simulink library "MAN_Library"  (R2023a)
settings: Solver=ode45  StartTime=0.0  StopTime=10.0  RelTol=1e-3  EnableMultiTasking=on
undefined symbols (not defined in the file): EventID
libraries: $bdroot x33, simulink_need_slupdate x1
(part 2 of 2)

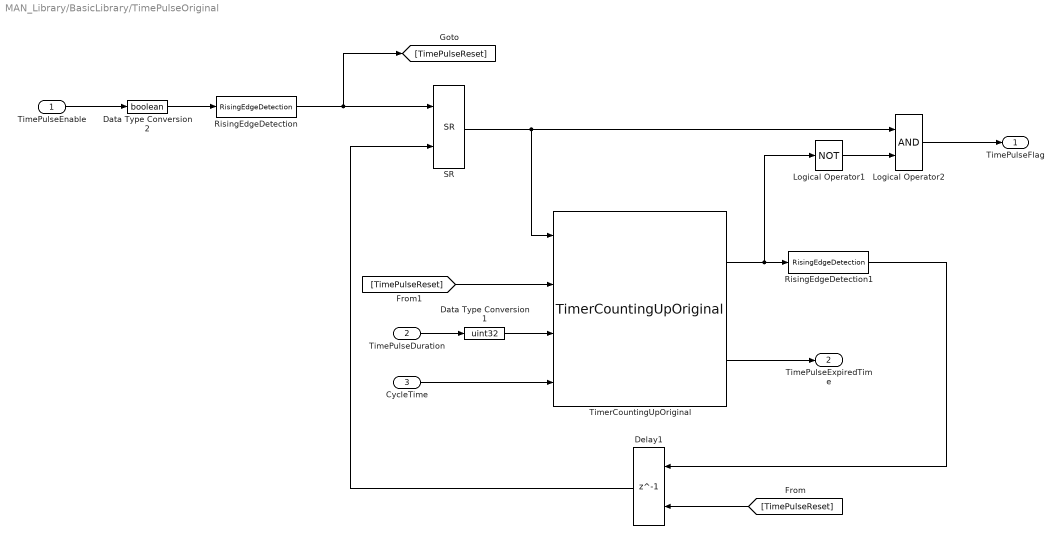
== system MAN_Library/BasicLibrary/TimePulseOriginal ==
  TimePulseEnable : Inport
  TimePulseDuration : Inport  Port=2
  CycleTime : Inport  Port=3
  Data Type Conversion1 : DataTypeConversion  OutDataTypeStr=uint32  SaturateOnIntegerOverflow=off  RndMeth=Floor
  Data Type Conversion2 : DataTypeConversion  OutDataTypeStr=boolean  SaturateOnIntegerOverflow=off  RndMeth=Floor
  Delay1 : Delay  DelayLength=1  InitialCondition=0  ExternalReset=Rising
      settings: InputPortMap=u0,r5
  Logical Operator1 : Logic  Operator=NOT  AllPortsSameDT=off  OutDataTypeStr=boolean
  Logical Operator2 : Logic  AllPortsSameDT=off  OutDataTypeStr=boolean
  RisingEdgeDetection : $bdroot/RisingEdgeDetection  SystemSampleTime=-1  VariantActivationTime=update diagram  Latency=0  AutoFrameSizeCalculation=off
  RisingEdgeDetection1 : $bdroot/RisingEdgeDetection  SystemSampleTime=-1  VariantActivationTime=update diagram  Latency=0  AutoFrameSizeCalculation=off
  SR : $bdroot/SR  SystemSampleTime=-1  VariantActivationTime=update diagram  Latency=0  AutoFrameSizeCalculation=off
  TimerCountingUpOriginal : $bdroot/BasicLibrary/TimerCountingUpOriginal  SystemSampleTime=-1  VariantActivationTime=update diagram  Latency=0  AutoFrameSizeCalculation=off
  TimePulseFlag : Outport
  TimePulseExpiredTime : Outport  Port=2
  wires:
  TimerCountingUpOriginal/2 -> TimePulseExpiredTime/1
  TimePulseDuration/1 -> Data Type Conversion1/1
  TimePulseEnable/1 -> Data Type Conversion2/1
  SR/1 -> TimerCountingUpOriginal/1, Logical Operator2/1
  TimerCountingUpOriginal/1 -> Logical Operator1/1, RisingEdgeDetection1/1
  RisingEdgeDetection1/1 -> Delay1/1
  Logical Operator2/1 -> TimePulseFlag/1
  Logical Operator1/1 -> Logical Operator2/2
  Data Type Conversion2/1 -> RisingEdgeDetection/1
  Data Type Conversion1/1 -> TimerCountingUpOriginal/3
  RisingEdgeDetection/1 -> [TimePulseReset], SR/1
  [TimePulseReset] -> Delay1/2
  [TimePulseReset] -> TimerCountingUpOriginal/2
  Delay1/1 -> SR/2
  CycleTime/1 -> TimerCountingUpOriginal/4

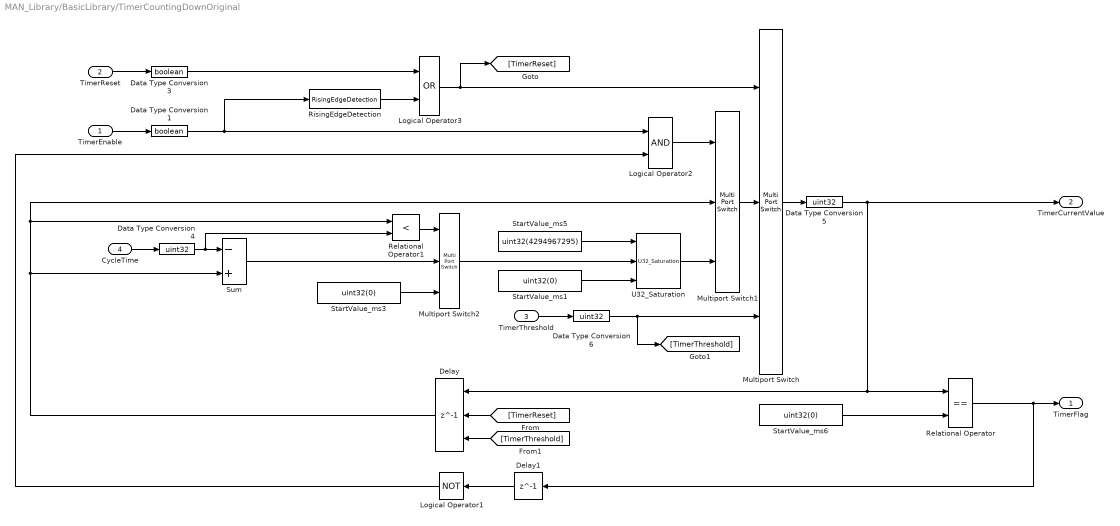
== system MAN_Library/BasicLibrary/TimerCountingDownOriginal ==
  TimerEnable : Inport
  TimerReset : Inport  Port=2
  TimerThreshold : Inport  Port=3
  CycleTime : Inport  Port=4
  Data Type Conversion1 : DataTypeConversion  OutDataTypeStr=boolean  SaturateOnIntegerOverflow=off  RndMeth=Floor
  Data Type Conversion3 : DataTypeConversion  OutDataTypeStr=boolean  SaturateOnIntegerOverflow=off  RndMeth=Floor
  Data Type Conversion4 : DataTypeConversion  OutDataTypeStr=uint32  SaturateOnIntegerOverflow=off  RndMeth=Floor
  Data Type Conversion5 : DataTypeConversion  OutDataTypeStr=uint32  SaturateOnIntegerOverflow=off  RndMeth=Floor
  Data Type Conversion6 : DataTypeConversion  OutDataTypeStr=uint32  SaturateOnIntegerOverflow=off  RndMeth=Floor
  Delay : Delay  DelayLength=1  InitialConditionSource=Input port  InitialCondition=0  ExternalReset=Rising
      settings: InputPortMap=u0,r5,p4
  Delay1 : Delay  DelayLength=1  InitialCondition=0
  Logical Operator1 : Logic  Operator=NOT  AllPortsSameDT=off  OutDataTypeStr=boolean
  Logical Operator2 : Logic  AllPortsSameDT=off  OutDataTypeStr=boolean
  Logical Operator3 : Logic  Operator=OR  AllPortsSameDT=off  OutDataTypeStr=boolean
  Multiport Switch : MultiPortSwitch  DataPortOrder=Zero-based contiguous  Inputs=2  zeroidx=on  SaturateOnIntegerOverflow=off  InputSameDT=off
  Multiport Switch1 : MultiPortSwitch  DataPortOrder=Zero-based contiguous  Inputs=2  zeroidx=on  SaturateOnIntegerOverflow=off  InputSameDT=off
  Multiport Switch2 : MultiPortSwitch  DataPortOrder=Zero-based contiguous  Inputs=2  zeroidx=on  SaturateOnIntegerOverflow=off  InputSameDT=off
  Relational Operator : RelationalOperator  Operator===  OutDataTypeStr=boolean  InputSameDT=off
  Relational Operator1 : RelationalOperator  Operator=<  OutDataTypeStr=boolean  InputSameDT=off
  RisingEdgeDetection : $bdroot/RisingEdgeDetection  SystemSampleTime=-1  VariantActivationTime=update diagram  Latency=0  AutoFrameSizeCalculation=off
  StartValue_ms1 : Constant  Value=uint32(0)  OutDataTypeStr=uint32
  StartValue_ms3 : Constant  Value=uint32(0)  OutDataTypeStr=uint32
  StartValue_ms5 : Constant  Value=uint32(4294967295)  OutDataTypeStr=uint32
  StartValue_ms6 : Constant  Value=uint32(0)  OutDataTypeStr=uint32
  Sum : Sum  Inputs=-+
  U32_Saturation : $bdroot/U32_Saturation  SystemSampleTime=-1  VariantActivationTime=update diagram  Latency=0  AutoFrameSizeCalculation=off
  TimerFlag : Outport
  TimerCurrentValue : Outport  Port=2
  wires:
  [TimerReset] -> Delay/2
  TimerThreshold/1 -> Data Type Conversion6/1
  Multiport Switch1/1 -> Multiport Switch/2
  Relational Operator/1 -> Delay1/1, TimerFlag/1
  Multiport Switch/1 -> Data Type Conversion5/1
  Data Type Conversion1/1 -> RisingEdgeDetection/1, Logical Operator2/1
  Data Type Conversion5/1 -> Relational Operator/1, Delay/1, TimerCurrentValue/1
  Logical Operator2/1 -> Multiport Switch1/1
  Logical Operator1/1 -> Logical Operator2/2
  U32_Saturation/1 -> Multiport Switch1/3
  Delay1/1 -> Logical Operator1/1
  StartValue_ms5/1 -> U32_Saturation/1
  Delay/1 -> Relational Operator1/1, Multiport Switch1/2, Sum/2
  Relational Operator1/1 -> Multiport Switch2/1
  Sum/1 -> Multiport Switch2/2
  Multiport Switch2/1 -> U32_Saturation/2
  StartValue_ms1/1 -> U32_Saturation/3
  CycleTime/1 -> Data Type Conversion4/1
  StartValue_ms6/1 -> Relational Operator/2
  TimerEnable/1 -> Data Type Conversion1/1
  Data Type Conversion6/1 -> [TimerThreshold], Multiport Switch/3
  Data Type Conversion4/1 -> Relational Operator1/2, Sum/1
  [TimerThreshold] -> Delay/3
  Logical Operator3/1 -> Multiport Switch/1, [TimerReset]
  Data Type Conversion3/1 -> Logical Operator3/1
  RisingEdgeDetection/1 -> Logical Operator3/2
  TimerReset/1 -> Data Type Conversion3/1
  StartValue_ms3/1 -> Multiport Switch2/3

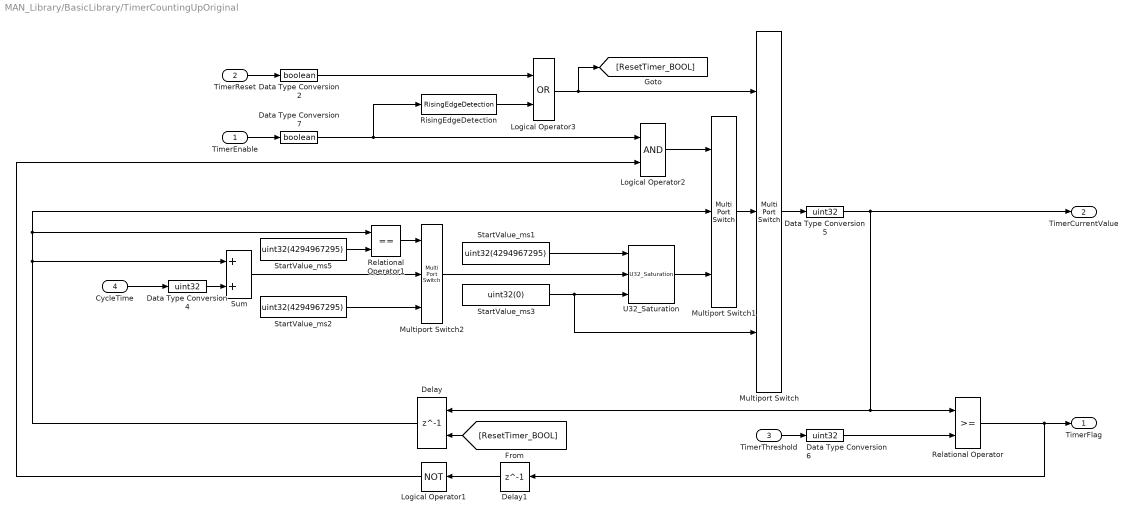
== system MAN_Library/BasicLibrary/TimerCountingUpOriginal ==
  TimerEnable : Inport
  TimerReset : Inport  Port=2
  TimerThreshold : Inport  Port=3
  CycleTime : Inport  Port=4
  Data Type Conversion2 : DataTypeConversion  OutDataTypeStr=boolean  SaturateOnIntegerOverflow=off  RndMeth=Floor
  Data Type Conversion4 : DataTypeConversion  OutDataTypeStr=uint32  SaturateOnIntegerOverflow=off  RndMeth=Floor
  Data Type Conversion5 : DataTypeConversion  OutDataTypeStr=uint32  SaturateOnIntegerOverflow=off  RndMeth=Floor
  Data Type Conversion6 : DataTypeConversion  OutDataTypeStr=uint32  SaturateOnIntegerOverflow=off  RndMeth=Floor
  Data Type Conversion7 : DataTypeConversion  OutDataTypeStr=boolean  SaturateOnIntegerOverflow=off  RndMeth=Floor
  Delay : Delay  DelayLength=1  InitialCondition=0  ExternalReset=Rising
      settings: InputPortMap=u0,r5
  Delay1 : Delay  DelayLength=1  InitialCondition=0
  Logical Operator1 : Logic  Operator=NOT  AllPortsSameDT=off  OutDataTypeStr=boolean
  Logical Operator2 : Logic  AllPortsSameDT=off  OutDataTypeStr=boolean
  Logical Operator3 : Logic  Operator=OR  AllPortsSameDT=off  OutDataTypeStr=boolean
  Multiport Switch : MultiPortSwitch  DataPortOrder=Zero-based contiguous  Inputs=2  zeroidx=on  SaturateOnIntegerOverflow=off  InputSameDT=off
  Multiport Switch1 : MultiPortSwitch  DataPortOrder=Zero-based contiguous  Inputs=2  zeroidx=on  SaturateOnIntegerOverflow=off  InputSameDT=off
  Multiport Switch2 : MultiPortSwitch  DataPortOrder=Zero-based contiguous  Inputs=2  zeroidx=on  SaturateOnIntegerOverflow=off  InputSameDT=off
  Relational Operator : RelationalOperator  OutDataTypeStr=boolean  InputSameDT=off
  Relational Operator1 : RelationalOperator  Operator===  OutDataTypeStr=boolean  InputSameDT=off
  RisingEdgeDetection : $bdroot/RisingEdgeDetection  SystemSampleTime=-1  VariantActivationTime=update diagram  Latency=0  AutoFrameSizeCalculation=off
  StartValue_ms1 : Constant  Value=uint32(4294967295)  OutDataTypeStr=uint32
  StartValue_ms2 : Constant  Value=uint32(4294967295)  OutDataTypeStr=uint32
  StartValue_ms3 : Constant  Value=uint32(0)  OutDataTypeStr=uint32
  StartValue_ms5 : Constant  Value=uint32(4294967295)  OutDataTypeStr=uint32
  Sum : Sum
  U32_Saturation : $bdroot/U32_Saturation  SystemSampleTime=-1  VariantActivationTime=update diagram  Latency=0  AutoFrameSizeCalculation=off
  TimerFlag : Outport
  TimerCurrentValue : Outport  Port=2
  wires:
  [ResetTimer_BOOL] -> Delay/2
  TimerThreshold/1 -> Data Type Conversion6/1
  Multiport Switch1/1 -> Multiport Switch/2
  Relational Operator/1 -> Delay1/1, TimerFlag/1
  Multiport Switch/1 -> Data Type Conversion5/1
  Data Type Conversion7/1 -> RisingEdgeDetection/1, Logical Operator2/1
  Data Type Conversion5/1 -> Relational Operator/1, Delay/1, TimerCurrentValue/1
  Logical Operator2/1 -> Multiport Switch1/1
  Logical Operator1/1 -> Logical Operator2/2
  U32_Saturation/1 -> Multiport Switch1/3
  Delay1/1 -> Logical Operator1/1
  StartValue_ms1/1 -> U32_Saturation/1
  Logical Operator3/1 -> [ResetTimer_BOOL], Multiport Switch/1
  StartValue_ms5/1 -> Relational Operator1/2
  Delay/1 -> Sum/1, Relational Operator1/1, Multiport Switch1/2
  Relational Operator1/1 -> Multiport Switch2/1
  StartValue_ms2/1 -> Multiport Switch2/3
  Sum/1 -> Multiport Switch2/2
  Multiport Switch2/1 -> U32_Saturation/2
  StartValue_ms3/1 -> Multiport Switch/3, U32_Saturation/3
  Data Type Conversion4/1 -> Sum/2
  Data Type Conversion6/1 -> Relational Operator/2
  TimerEnable/1 -> Data Type Conversion7/1
  TimerReset/1 -> Data Type Conversion2/1
  RisingEdgeDetection/1 -> Logical Operator3/2
  Data Type Conversion2/1 -> Logical Operator3/1
  CycleTime/1 -> Data Type Conversion4/1

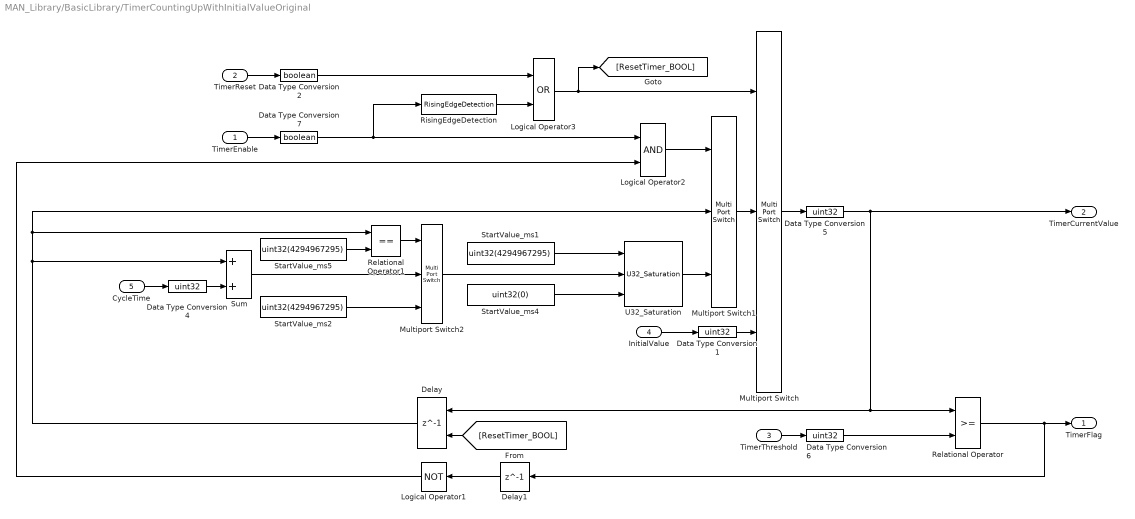
== system MAN_Library/BasicLibrary/TimerCountingUpWithInitialValueOriginal ==
  TimerEnable : Inport
  TimerReset : Inport  Port=2
  TimerThreshold : Inport  Port=3
  InitialValue : Inport  Port=4
  CycleTime : Inport  Port=5
  Data Type Conversion{1,4..6} (4 alike) : DataTypeConversion  OutDataTypeStr=uint32  SaturateOnIntegerOverflow=off  RndMeth=Floor
  Data Type Conversion2 : DataTypeConversion  OutDataTypeStr=boolean  SaturateOnIntegerOverflow=off  RndMeth=Floor
  Data Type Conversion7 : DataTypeConversion  OutDataTypeStr=boolean  SaturateOnIntegerOverflow=off  RndMeth=Floor
  Delay : Delay  DelayLength=1  InitialCondition=0  ExternalReset=Rising
      settings: InputPortMap=u0,r5
  Delay1 : Delay  DelayLength=1  InitialCondition=0
  Logical Operator1 : Logic  Operator=NOT  AllPortsSameDT=off  OutDataTypeStr=boolean
  Logical Operator2 : Logic  AllPortsSameDT=off  OutDataTypeStr=boolean
  Logical Operator3 : Logic  Operator=OR  AllPortsSameDT=off  OutDataTypeStr=boolean
  Multiport Switch : MultiPortSwitch  DataPortOrder=Zero-based contiguous  Inputs=2  zeroidx=on  SaturateOnIntegerOverflow=off  InputSameDT=off
  Multiport Switch1 : MultiPortSwitch  DataPortOrder=Zero-based contiguous  Inputs=2  zeroidx=on  SaturateOnIntegerOverflow=off  InputSameDT=off
  Multiport Switch2 : MultiPortSwitch  DataPortOrder=Zero-based contiguous  Inputs=2  zeroidx=on  SaturateOnIntegerOverflow=off  InputSameDT=off
  Relational Operator : RelationalOperator  OutDataTypeStr=boolean  InputSameDT=off
  Relational Operator1 : RelationalOperator  Operator===  OutDataTypeStr=boolean  InputSameDT=off
  RisingEdgeDetection : $bdroot/RisingEdgeDetection  SystemSampleTime=-1  VariantActivationTime=update diagram  Latency=0  AutoFrameSizeCalculation=off
  StartValue_ms1 : Constant  Value=uint32(4294967295)  OutDataTypeStr=uint32
  StartValue_ms2 : Constant  Value=uint32(4294967295)  OutDataTypeStr=uint32
  StartValue_ms4 : Constant  Value=uint32(0)  OutDataTypeStr=uint32
  StartValue_ms5 : Constant  Value=uint32(4294967295)  OutDataTypeStr=uint32
  Sum : Sum
  U32_Saturation : $bdroot/U32_Saturation  SystemSampleTime=-1  VariantActivationTime=update diagram  Latency=0  AutoFrameSizeCalculation=off
  TimerFlag : Outport
  TimerCurrentValue : Outport  Port=2
  wires:
  [ResetTimer_BOOL] -> Delay/2
  TimerThreshold/1 -> Data Type Conversion6/1
  Multiport Switch1/1 -> Multiport Switch/2
  Relational Operator/1 -> Delay1/1, TimerFlag/1
  Multiport Switch/1 -> Data Type Conversion5/1
  Data Type Conversion7/1 -> RisingEdgeDetection/1, Logical Operator2/1
  Data Type Conversion5/1 -> Relational Operator/1, Delay/1, TimerCurrentValue/1
  Logical Operator2/1 -> Multiport Switch1/1
  Logical Operator1/1 -> Logical Operator2/2
  U32_Saturation/1 -> Multiport Switch1/3
  Delay1/1 -> Logical Operator1/1
  StartValue_ms1/1 -> U32_Saturation/1
  Logical Operator3/1 -> [ResetTimer_BOOL], Multiport Switch/1
  StartValue_ms5/1 -> Relational Operator1/2
  Delay/1 -> Sum/1, Relational Operator1/1, Multiport Switch1/2
  Relational Operator1/1 -> Multiport Switch2/1
  StartValue_ms2/1 -> Multiport Switch2/3
  Sum/1 -> Multiport Switch2/2
  Multiport Switch2/1 -> U32_Saturation/2
  StartValue_ms4/1 -> U32_Saturation/3
  Data Type Conversion4/1 -> Sum/2
  CycleTime/1 -> Data Type Conversion4/1
  Data Type Conversion6/1 -> Relational Operator/2
  TimerEnable/1 -> Data Type Conversion7/1
  TimerReset/1 -> Data Type Conversion2/1
  RisingEdgeDetection/1 -> Logical Operator3/2
  Data Type Conversion2/1 -> Logical Operator3/1
  InitialValue/1 -> Data Type Conversion1/1
  Data Type Conversion1/1 -> Multiport Switch/3

== system MAN_Library/BasicLibrary/TurnOffDelayOriginal ==
  TurnOffDelayEnable : Inport
  TurnOffDelayThreshold : Inport  Port=2
  CycleTime : Inport  Port=3
  Data Type Conversion1 : DataTypeConversion  OutDataTypeStr=uint32  SaturateOnIntegerOverflow=off  RndMeth=Floor
  Data Type Conversion2 : DataTypeConversion  OutDataTypeStr=boolean  SaturateOnIntegerOverflow=off  RndMeth=Floor
  Data Type Conversion3 : DataTypeConversion  OutDataTypeStr=uint32  SaturateOnIntegerOverflow=off  RndMeth=Floor
  FallingEdgeDetection : $bdroot/FallingEdgeDetection  SystemSampleTime=-1  VariantActivationTime=update diagram  Latency=0  AutoFrameSizeCalculation=off
  Logical Operator2 : Logic  Operator=OR  AllPortsSameDT=off  OutDataTypeStr=boolean
  TimePulseOriginal : $bdroot/BasicLibrary/TimePulseOriginal  SystemSampleTime=-1  VariantActivationTime=update diagram  Latency=0  AutoFrameSizeCalculation=off
  TurnOffDelayFlag : Outport
  TurnOffDelayExpiredTime : Outport  Port=2
  wires:
  TurnOffDelayEnable/1 -> Data Type Conversion2/1
  Data Type Conversion2/1 -> Logical Operator2/1, FallingEdgeDetection/1
  TimePulseOriginal/1 -> Logical Operator2/2
  Logical Operator2/1 -> TurnOffDelayFlag/1
  TimePulseOriginal/2 -> Data Type Conversion3/1
  FallingEdgeDetection/1 -> TimePulseOriginal/1
  TurnOffDelayThreshold/1 -> Data Type Conversion1/1
  Data Type Conversion1/1 -> TimePulseOriginal/2
  Data Type Conversion3/1 -> TurnOffDelayExpiredTime/1
  CycleTime/1 -> TimePulseOriginal/3

== system MAN_Library/BasicLibrary/TurnOnDelayOriginal ==
  TurnOnDelayEnable : Inport
  TurnOnDelayThreshold : Inport  Port=2
  CycleTime : Inport  Port=3
  Data Type Conversion1 : DataTypeConversion  OutDataTypeStr=uint32  SaturateOnIntegerOverflow=off  RndMeth=Floor
  Data Type Conversion2 : DataTypeConversion  OutDataTypeStr=boolean  SaturateOnIntegerOverflow=off  RndMeth=Floor
  Logical Operator1 : Logic  Operator=NOT  AllPortsSameDT=off  OutDataTypeStr=boolean
  Logical Operator2 : Logic  AllPortsSameDT=off  OutDataTypeStr=boolean
  RisingEdgeDetection : $bdroot/RisingEdgeDetection  SystemSampleTime=-1  VariantActivationTime=update diagram  Latency=0  AutoFrameSizeCalculation=off
  TimePulseOriginal : $bdroot/BasicLibrary/TimePulseOriginal  SystemSampleTime=-1  VariantActivationTime=update diagram  Latency=0  AutoFrameSizeCalculation=off
  TurnOnDelayFlag : Outport
  TurnOnDelayExpiredTime : Outport  Port=2
  wires:
  Data Type Conversion2/1 -> Logical Operator2/1, RisingEdgeDetection/1
  TurnOnDelayEnable/1 -> Data Type Conversion2/1
  TurnOnDelayThreshold/1 -> Data Type Conversion1/1
  Data Type Conversion1/1 -> TimePulseOriginal/2
  RisingEdgeDetection/1 -> TimePulseOriginal/1
  TimePulseOriginal/2 -> TurnOnDelayExpiredTime/1
  Logical Operator1/1 -> Logical Operator2/2
  TimePulseOriginal/1 -> Logical Operator1/1
  Logical Operator2/1 -> TurnOnDelayFlag/1
  CycleTime/1 -> TimePulseOriginal/3

== system MAN_Library/Dem_SetEventStatus/Dem_SetEventStatus_Enable ==
  EventID : Inport
  EveSt : Inport  Port=2
  Enable : EnablePort
  Data Type Conversion : DataTypeConversion  SaturateOnIntegerOverflow=off  RndMeth=Floor
  Dem_SetEventStatus_Asw : S-Function  FunctionName=Dem_SetEventStatus_Asw_SF  SFunctionDeploymentMode=off  EnableBusSupport=off  mask(Legacy Function){SFunctionSpec=void Dem_SetEventStatus_Asw(uint16 u1, uint8 u2), ShowSpec=on}
      mask prompts: ShowSpec "Display function specification"
      mask help:
      | This block allows you to call the legacy functions specified by the following Legacy Code Tool definition:
      | def.SFunctionName = 'Dem_SetEventStatus_Asw_SF';
      | def.OutputFcnSpec = 'void Dem_SetEventStatus_Asw(uint16 u1, uint8 u2)';
      | def.HeaderFiles = {'Dem.h'};
      | def.SourceFiles = {'Dem.c'};
      mask Help: <p>This block was generated automatically by the Legacy Code Tool. For detailed help on this tool, call<a href="matlab:legacy_code('help')"> legacy_code('help')</a>.</p>
      mask Callback ShowSpec:
      | if strcmp(get_param(gcbh, 'ShowSpec'), 'on')
      |   set_param(gcbh, 'MaskDisplay', sprintf('fprintf(''%s'');', get_param(gcbh, 'SFunctionSpec')));
      | else
      |   set_param(gcbh, 'MaskDisplay', sprintf('fprintf(''%s'');', get_param(gcbh, 'FunctionName')));
      | end
      mask Display: fprintf('void Dem_SetEventStatus_Asw(uint16 u1, uint8 u2)');
  wires:
  EventID/1 -> Data Type Conversion/1
  EveSt/1 -> Dem_SetEventStatus_Asw/2
  Data Type Conversion/1 -> Dem_SetEventStatus_Asw/1
